simulink model "chapter5_P2"  (R2017a)
settings: Solver=ode1  StartTime=0.0  StopTime=inf  FixedStep=0.001  RelTol=1e-3  EnableMultiTasking=on
values from neighbouring files (symbols this model uses):
  A = [0 1 0 0;        a 0 0 0;        0 0 0 1;        0 0 0 0]    [ece486_finalproj1.m]
  B = [ 0; -bp; 0; br]    [ece486_finalproj1.m]
  C = [ 1 0 0 0; 0 0 1 0]    [ece486_finalproj1.m]
  K = place(A,B,[pls(1) pls(2) 0 real(pls(1)) ])    [ece486_finalproj1.m]
  L = L_hat    [ece486_finalproj1.m]
libraries: c6xlib x2
Description:
  | Real-Time Van der Pol Simulation
  | 
  | This demonstration shows a real-time version of the Simulink(R) Van der Pol
  | simulation demo. This model does not need any external signals, so it does
  | not need any data acquisition hardware or driver. This makes the model ideal
  | for first experiments with Real-Time Windows Target(TM), without need to
  | worry about proper I/O hardware configuration.
  | 
  | How to run this demo:
  | 
  |   1. Build the model using Tools -> Real-Time Workshop -> Build Model.
  |   2. Connect to the real-time code using Simulation -> Connect to target.
  |   3. Start the real-time execution using Simulation -> Start real-time code.
settings Model: SimulationMode=external  ExtModeTrigDuration=50000  Creator=Houska  LastModifiedBy=lwang114
settings DataIOCC: SaveFormat=Array  SignalLoggingSaveFormat=ModelDataLogs  SignalLoggingName=logsOut
settings OptimizationCC: ExpressionDepthLimit=2147483647  InitFltsAndDblsToZero=on  EfficientMapNaN2IntZero=off
settings DebuggingCC: UnderspecifiedInitializationDetection=Classic  MergeDetectMultiDrivingBlocksExec=none  SignalResolutionControl=TryResolveAllWithWarning  FcnCallInpInsideContextMsg=warning  StateNameClashWarn=warning  SFUnexpectedBacktrackingDiag=warning  SFNoUnconditionalDefaultTransitionDiag=warning  SFExecutionAtInitializationDiag=none
settings ModelReferenceCC: PropagateSignalLabelsOutOfModel=off
settings RTWCC: SystemTargetFile=sldrt.tlc  TemplateMakefile=sldrt.tmf  Description=Simulink Desktop Real-Time  RTWCompilerOptimization=on
settings CodeAppCC: MaxIdLength=95
settings SimulinkDesktopRealTimeCC: TargetPreCompLibLocation=C:\MATLABR2017a\toolbox\sldrt\lib\win64  TargetLangStandard=C89/C90 (ANSI)  SupportVariableSizeSignals=off
settings ConfigComp: CovMetricSettings=dw  CovHtmlReporting=on  CovSaveCumulativeToWorkspaceVar=on  CovSaveSingleToWorkspaceVar=on  CovExternalEMLEnable=off  CovSFcnEnable=off

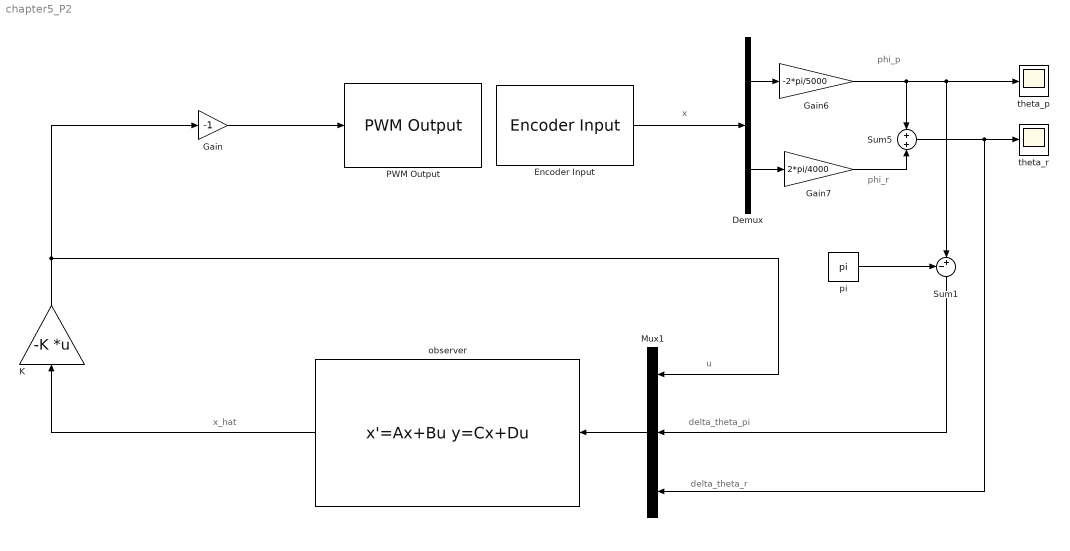
== system chapter5_P2 ==
  note: x_hat
  note: delta_theta_r
  note: delta_theta_pi
  note: u
  note: x
  note: phi_p
  note: phi_r
  Demux : Demux  Outputs=2
  Encoder Input : c6xlib/Encoder Input  baseAddr=0x378  channels=[0 1]  sampleTime=str2num(get_param(bdroot, 'FixedStep'))
  Gain : Gain  Gain=-1
  Gain6 : Gain  Gain=-2*pi/5000
  Gain7 : Gain  Gain=2*pi/4000
  K : Gain  Gain=-K  Multiplication=Matrix(K*u)
  Mux1 : Mux  Inputs=3
  PWM Output : c6xlib/PWM Output  baseAddr=0x378  channels=0  initialOutputs=0  finalOutputs=0  sampleTime=str2num(get_param(bdroot, 'FixedStep'))
  Sum1 : Sum  Inputs=-+|
  Sum5 : Sum
  observer : StateSpace  A=A-L*C  B=[B L]  C=eye(4)  D=zeros(4,3)  X0=0
  pi : Constant  Value=pi
  theta_p : Scope
  theta_r : Scope
  wires:
  Demux/1 -> Gain6/1
  Gain7/1 -> Sum5/2
  Demux/2 -> Gain7/1
  Encoder Input/1 -> Demux/1
  Gain6/1 -> Sum1/2, theta_p/1, Sum5/1
  Mux1/1 -> observer/1
  K/1 -> Gain/1, Mux1/1
  Sum1/1 -> Mux1/2
  Sum5/1 -> theta_r/1, Mux1/3
  Gain/1 -> PWM Output/1
  observer/1 -> K/1
  pi/1 -> Sum1/1
